simulink model "Q4section4"  (R2019a)
settings: Solver=VariableStepAuto  StartTime=0.0  StopTime=50  RelTol=1e-3
values from neighbouring files (symbols this model uses):
  c = 0.5    [q4.m]
  ca = 0.1    [q4.m]
  J = 0.07    [q4.m]
  Kb = Kt    (= 0.46)    [q4.m]
  Kt = 0.46    [q4.m]
  l = 0.3    [q4.m]
  L = 0    [q4.m]
  m = 0.8    [q4.m]
  N = 3    [q4.m]
  n = 0.95    [q4.m]
  R = 0.76    [q4.m]
libraries: cstblocks x1
settings Model: Creator=Nir Lalum  LastModifiedBy=Nir Lalum

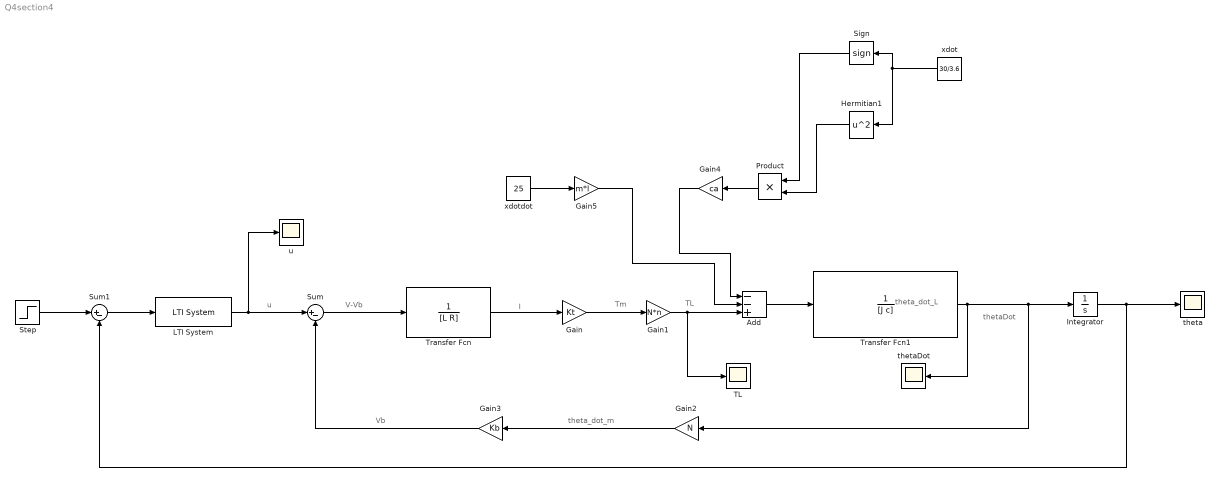
== system Q4section4 ==
  note: thetaDot
  note: u
  note: Vb
  note: theta_dot_m
  note: theta_dot_L
  note: TL
  note: Tm
  note: I
  note: V-Vb
  Add : Sum  Inputs=--+
  Gain : Gain  Gain=Kt
  Gain1 : Gain  Gain=N*n
  Gain2 : Gain  Gain=N
  Gain3 : Gain  Gain=Kb
  Gain4 : Gain  Gain=ca
  Gain5 : Gain  Gain=m*l
  Hermitian1 : Math  Operator=square  SaturateOnIntegerOverflow=on
  Integrator : Integrator
  LTI System : cstblocks/LTI System  sys=C_PI  IC=[]
  Product : Product
  Sign : Signum
  Step : Step  Time=0  After=7.3  SampleTime=0
  Sum : Sum  Inputs=|+-
  Sum1 : Sum  Inputs=|+-
  TL : Scope
  Transfer Fcn : TransferFcn  Denominator=[L R]
  Transfer Fcn1 : TransferFcn  Denominator=[J c]
  "theta " : Scope
  thetaDot : Scope
  u : Scope
  xdot : Constant  Value=30/3.6
  xdotdot : Constant  Value=25
  wires:
  Sum/1 -> Transfer Fcn/1
  Transfer Fcn/1 -> Gain/1
  Gain/1 -> Gain1/1
  Transfer Fcn1/1 -> thetaDot/1, Gain2/1, Integrator/1
  Integrator/1 -> Sum1/2, "theta "/1
  Gain2/1 -> Gain3/1
  Gain3/1 -> Sum/2
  Product/1 -> Gain4/1
  xdot/1 -> Hermitian1/1, Sign/1
  Sign/1 -> Product/1
  Hermitian1/1 -> Product/2
  xdotdot/1 -> Gain5/1
  Step/1 -> Sum1/1
  Sum1/1 -> LTI System/1
  Gain1/1 -> TL/1, Add/3
  Gain5/1 -> Add/2
  Gain4/1 -> Add/1
  Add/1 -> Transfer Fcn1/1
  LTI System/1 -> u/1, Sum/1
